simulink model "PSKs_Lab"  (R2021a)
settings: Solver=VariableStepAuto  StartTime=0.0  StopTime=50/Rb  FixedStep=1e-8  RelTol=1e-3
values from neighbouring files (symbols this model uses):
  Amplitud = 1    [Sinc_PSKm.m]
  Ancho_banda_minimo = Rb / 2    (= 500)    [Sinc_PSKm.m]
  Att_pot_Canal = 10^(Att_dB / 10)    [Sinc_PSKm.m]
  Att_Volt_Canal = 10^(Att_dB / 20)    [Sinc_PSKm.m]
  b = 0.6    [Sinc_PSKm.m]
  C = 1e-6    (= 1e-06)    [Sinc_PSKm.m]
  Frec_port = 100 * Rb    (= 100000)    [Sinc_PSKm.m]
  Kv = 1E5    (= 100000)    [Sinc_PSKm.m]
  Pot_Ruido = 2*eta * Ancho_banda_minimo    [Sinc_PSKm.m]
  R1 = Kp * Kv / (wn^2 * C)    (= 98.7654320988)    [Sinc_PSKm.m]
  R2 = 2 * zita / (wn * C)    (= 53.3333333333)    [Sinc_PSKm.m]
  Rb = 1000    [Sinc_PSKm.m]
  Retraso_Canal = Long_Canal / C_canal+0.5/Frec_port    (= 3.83333333333e-05)    [Sinc_PSKm.m]
  Tb = 1 / Rb    (= 0.001)    [Sinc_PSKm.m]
  Umbral = 0    [Sinc_PSKm.m]
libraries: dspsigops x4, dsparch4 x3, simulink_extras x3, simulink x2, commsynccomp2 x2, powerlib_extras x2, commrandsrc3 x1
settings Model: Creator=PedroPablo  LastModifiedBy=ppbot
settings SolverCC: AlgebraicLoopSolver=TrustRegion
settings DebuggingCC: SFMachineParentedDataDiag=warning

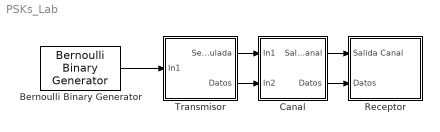
== system PSKs_Lab ==
  Bernoulli Binary Generator : commrandsrc3/Bernoulli Binary Generator  ProbabilityOfZero=0.5  SeedSource=Parameter  Seed=61  SampleTime=1/Rb  SamplesPerFrame=1  OutputDataType=double  SimulateUsing=Interpreted execution
  Canal : Subsystem
  Receptor : Subsystem
  Transmisor : Subsystem
  wires:
  Bernoulli Binary Generator/1 -> Transmisor/1(In1)
  Transmisor/1(Señal modulada) -> Canal/1(In1)
  Transmisor/2(Datos) -> Canal/2(In2)
  Canal/1(Salida Canal) -> Receptor/1(Salida Canal)
  Canal/2(Datos) -> Receptor/2(Datos)

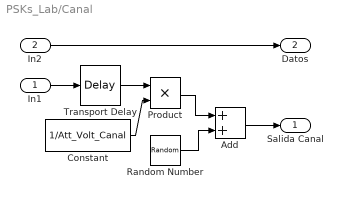
== system PSKs_Lab/Canal ==
  In1 : Inport
  In2 : Inport  Port=2
  Add : Sum
  Constant : Constant  Value=1/Att_Volt_Canal
  Product : Product
  Random Number : RandomNumber  Variance=Pot_Ruido  SampleTime=1/(10000*Rb)
  Transport Delay : TransportDelay  DelayTime=Retraso_Canal
  Salida Canal : Outport
  Datos : Outport  Port=2
  wires:
  In2/1 -> Datos/1
  Product/1 -> Add/1
  Add/1 -> Salida Canal/1
  Constant/1 -> Product/2
  In1/1 -> Transport Delay/1
  Random Number/1 -> Add/2
  Transport Delay/1 -> Product/1

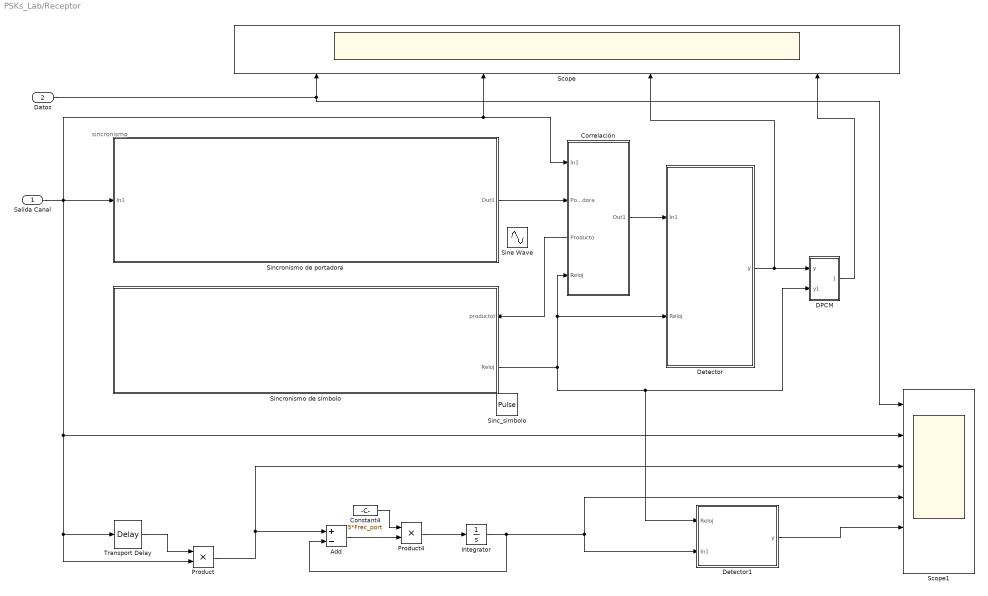
== system PSKs_Lab/Receptor ==
  note: sincronismo
  Salida Canal : Inport
  Datos : Inport  Port=2
  Add : Sum  Inputs=+-
  Constant4 : Constant  Value=5*Frec_port
  Correlación : Subsystem
      settings: PortSchema="{\"entries\":[{\"content\":{\"sides\":[{\"content\":{\"connectorIds\":[\"In1\",\"In2\",\"Out2\",\"In3\"]},\"type\":\"ConnectorPlacement.EquallySpacedRectSide\",\"uuid\":\"9c9ed9ca-e8ca-44c2-a659-85a067b2e2ab\"},{\"content\":{\"connectorIds\":[\"Out1\"],\"side\":\"RIGHT\"},\"type\":\"ConnectorPlacement.EquallySpacedRectSide\",\"uuid\":\"749548a8-d339-4a18-8c47-3529cad88115\"},{\"content\":{\"connectorIds\":[],\"side\":\"TOP\"},\"type\":\"ConnectorPlacement.EquallySpacedRectSide\",\"uuid\":\"502cb8ca-7e6c-4f6d-9acf-9edc021ca5d9\"},{\"content\":{\"connectorIds\":[],\"side\":\"BOTTOM\"},\"type\":\"ConnectorPlacement.EquallySpacedRectSide\",\"uuid\":\"343f95ab-8b43-4ca2-96bf-a55a52c277fe\"}]},\"type\":\"ConnectorPlacement.EquallySpacedConnector\",\"uuid\":\"c50381c4-8798-4039-a023-6424d6fa731c\"}],\"packageUris\":[\"http://schema.mathworks.com/mf0/Connector/R2020b\"],\"version\":\"1.0\"}"
  DPCM : Subsystem
  Detector : Subsystem
  Detector1 : Subsystem
  Integrator : Integrator
  Product : Product
  Product4 : Product
  Scope : Scope  NumInputPorts=4
  Scope1 : Scope  NumInputPorts=6
  Sinc_simbolo : DiscretePulseGenerator  PulseType=Time based  Amplitude=Amplitud  Period=1/Rb  PulseWidth=50
  Sincronismo de portadora : Subsystem
  Sincronismo de símbolo : Subsystem
      settings: PortSchema="{\"entries\":[{\"content\":{\"sides\":[{\"content\":{\"connectorIds\":[]},\"type\":\"ConnectorPlacement.EquallySpacedRectSide\",\"uuid\":\"93994b0c-b2cb-4331-9695-4cda4bbb6019\"},{\"content\":{\"connectorIds\":[\"In1\",\"Out1\"],\"side\":\"RIGHT\"},\"type\":\"ConnectorPlacement.EquallySpacedRectSide\",\"uuid\":\"b8064540-0ede-4985-840d-1e59709fa35b\"},{\"content\":{\"connectorIds\":[],\"side\":\"TOP\"},\"type\":\"ConnectorPlacement.EquallySpacedRectSide\",\"uuid\":\"0f7e7988-f1a5-40c2-b0ce-e0a51a477c0a\"}]},\"type\":\"ConnectorPlacement.EquallySpacedConnector\",\"uuid\":\"3553a0bb-71d1-453e-9ff3-b6164d2735c0\"}],\"packageUris\":[\"http://schema.mathworks.com/mf0/Connector/R2020b\"],\"version\":\"1.0\"}"
  Sine Wave : Sin  Amplitude=Amplitud/Att_Volt_Canal  Frequency=2*pi*Frec_port  SampleTime=0
  Transport Delay : TransportDelay  DelayTime=Tb
  wires:
  Datos/1 -> Scope/1, Scope1/1
  Correlación/1(Out1) -> Detector/1(In1)
  Detector/1(y) -> Scope/3, DPCM/1(y)
  Sincronismo de portadora/1(Out1) -> Correlación/2(Portadora)
  Sincronismo de símbolo/1(Reloj) -> Correlación/3(Reloj), Detector/2(Reloj), Detector1/1(Reloj), DPCM/2(y1)
  Salida Canal/1 -> Transport Delay/1, Product/2, Scope1/2, Correlación/1(In1), Scope/2, Sincronismo de portadora/1(In1)
  Correlación/2(Producto) -> Sincronismo de símbolo/1(productol)
  DPCM/1(Out1) -> Scope/4
  Transport Delay/1 -> Product/1
  Product/1 -> Scope1/3, Add/1
  Constant4/1 -> Product4/1
  Product4/1 -> Integrator/1
  Integrator/1 -> Add/2, Detector1/2(In1), Scope1/4
  Add/1 -> Product4/2
  Detector1/1(y) -> Scope1/5

== system PSKs_Lab/Transmisor ==
  In1 : Inport
  Analog Filter Design : dsparch4/Analog Filter Design  method=Butterworth  filttype=Bandpass  N=2  Wlo=2*pi*(Frec_port - 2*Ancho_banda_minimo)  Whi=2*pi*(Frec_port + 2*Ancho_banda_minimo)  Rp=2  Rs=40
  Modulador : Subsystem
  Señal modulada : Outport
  Datos : Outport  Port=2
  wires:
  In1/1 -> Modulador/1(In1), Datos/1
  Analog Filter Design/1 -> Señal modulada/1
  Modulador/1(Out1) -> Analog Filter Design/1

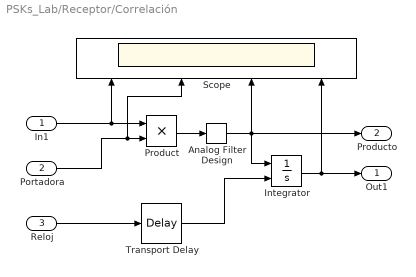
== system PSKs_Lab/Receptor/Correlación ==
  In1 : Inport
  Portadora : Inport  Port=2
  Reloj : Inport  Port=3
  Analog Filter Design : dsparch4/Analog Filter Design  method=Butterworth  filttype=Lowpass  N=8  Wlo=2*pi*Rb  Whi=80  Rp=2  Rs=40
  Integrator : Integrator  ExternalReset=rising
  Product : Product
  Scope : Scope  NumInputPorts=4
  Transport Delay : TransportDelay  DelayTime=1e-9
  Out1 : Outport
  Producto : Outport  Port=2
  wires:
  Transport Delay/1 -> Integrator/2
  In1/1 -> Product/1, Scope/1
  Integrator/1 -> Out1/1, Scope/4
  Reloj/1 -> Transport Delay/1
  Product/1 -> Analog Filter Design/1
  Portadora/1 -> Scope/2, Product/2
  Analog Filter Design/1 -> Integrator/1, Scope/3, Producto/1

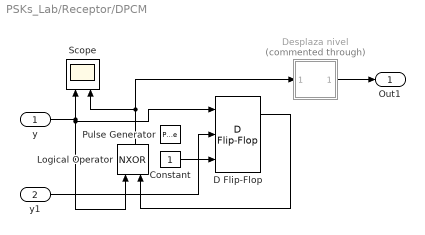
== system PSKs_Lab/Receptor/DPCM ==
  y : Inport
  y1 : Inport  Port=2
  Constant : Constant
  D Flip-Flop : simulink_extras/Flip Flops/D Flip-Flop
  Desplaza nivel : Subsystem  Commented=through
  Logical Operator : Logic  Operator=NXOR  AllPortsSameDT=off  OutDataTypeStr=boolean
  Pulse Generator : DiscretePulseGenerator  PulseType=Time based  Period=Tb
  Scope : Scope  NumInputPorts=2
  Out1 : Outport
  wires:
  Logical Operator/1 -> Desplaza nivel/1(In1), Scope/2
  D Flip-Flop/1 -> Logical Operator/2
  Constant/1 -> D Flip-Flop/3
  y/1 -> Scope/1, D Flip-Flop/1, Logical Operator/1
  Desplaza nivel/1(Out1) -> Out1/1
  y1/1 -> D Flip-Flop/2

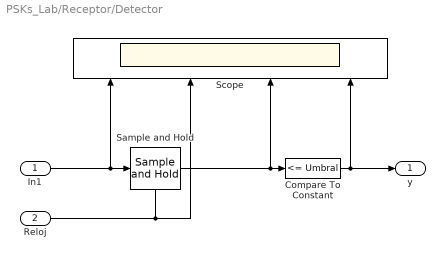
== system PSKs_Lab/Receptor/Detector ==
  In1 : Inport
  Reloj : Inport  Port=2
  Compare To Constant : simulink/Logic and Bit Operations/Compare To Constant  relop=<=  const=Umbral  OutDataTypeStr=boolean
  Sample and Hold : dspsigops/Sample and Hold  trig=Rising edge  initCond=0  latchinput=off
  Scope : Scope  NumInputPorts=4
  y : Outport
  wires:
  In1/1 -> Sample and Hold/1, Scope/1
  Compare To Constant/1 -> Scope/4, y/1
  Reloj/1 -> Scope/2, Sample and Hold/Trigger
  Sample and Hold/1 -> Scope/3, Compare To Constant/1

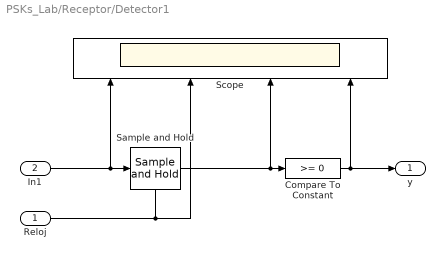
== system PSKs_Lab/Receptor/Detector1 ==
  Reloj : Inport
  In1 : Inport  Port=2
  Compare To Constant : simulink/Logic and Bit Operations/Compare To Constant  relop=>=  const=0  OutDataTypeStr=boolean
  Sample and Hold : dspsigops/Sample and Hold  trig=Rising edge  initCond=0  latchinput=off
  Scope : Scope  NumInputPorts=4
  y : Outport
  wires:
  In1/1 -> Sample and Hold/1, Scope/1
  Compare To Constant/1 -> Scope/4, y/1
  Reloj/1 -> Scope/2, Sample and Hold/Trigger
  Sample and Hold/1 -> Scope/3, Compare To Constant/1

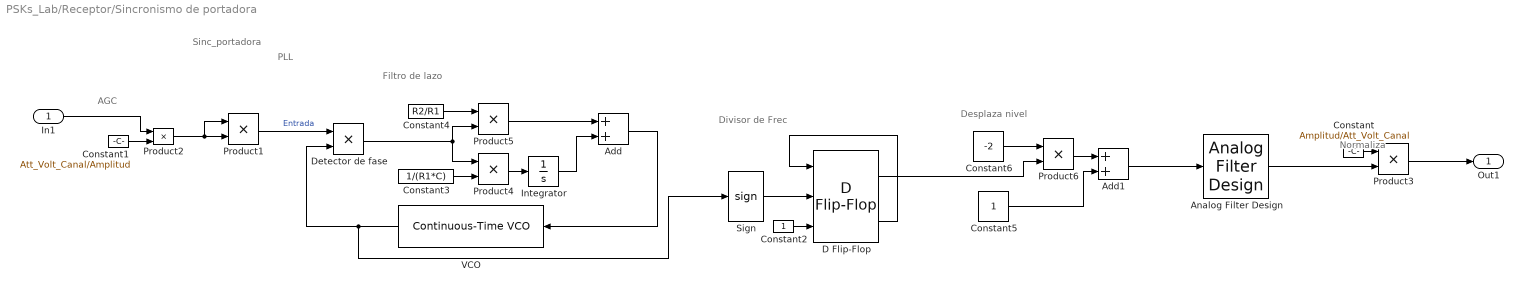
== system PSKs_Lab/Receptor/Sincronismo de portadora ==
  note: Desplaza nivel
  note: Filtro de lazo
  note: Divisor de Frec
  note: PLL
  note: Normaliza
  note: Sinc_portadora
  note: AGC
  In1 : Inport
  " VCO" : commsynccomp2/Continuous-Time VCO  Ac=1  Fc=2*Frec_port  Kc=Kv/(2*pi)  Ph=0
      settings: SourceProductBaseCode=CM
  Add : Sum
  Add1 : Sum
  Analog Filter Design : dsparch4/Analog Filter Design  method=Butterworth  filttype=Bandpass  N=2  Wlo=1.8*pi*Frec_port  Whi=2.2*pi*Frec_port  Rp=2  Rs=40
  Constant : Constant  Value=Amplitud/Att_Volt_Canal
  Constant1 : Constant  Value=Att_Volt_Canal/Amplitud
  Constant2 : Constant
  Constant3 : Constant  Value=1/(R1*C)
  Constant4 : Constant  Value=R2/R1
  Constant5 : Constant
  Constant6 : Constant  Value=-2
  D Flip-Flop : simulink_extras/Flip Flops/D Flip-Flop
  Detector de fase : Product
  Integrator : Integrator
  Product{1..6} (6 alike) : Product
  Sign : Signum
  Out1 : Outport
  wires:
  Product3/1 -> Out1/1
  In1/1 -> Product2/1
  Constant1/1 -> Product2/2
  Product2/1 -> Product1/1, Product1/2
  Constant/1 -> Product3/1
  Add1/1 -> Analog Filter Design/1
  Add/1 -> " VCO"/1
  Product1/1 -> Detector de fase/1  "Entrada"
  Sign/1 -> D Flip-Flop/2
  " VCO"/1 -> Detector de fase/2, Sign/1
  D Flip-Flop/2 -> D Flip-Flop/1
  Constant2/1 -> D Flip-Flop/3
  Constant4/1 -> Product5/1
  Product5/1 -> Add/1
  Detector de fase/1 -> Product5/2, Product4/1
  Product4/1 -> Integrator/1
  Integrator/1 -> Add/2
  Constant3/1 -> Product4/2
  Constant5/1 -> Add1/2
  Product6/1 -> Add1/1
  Constant6/1 -> Product6/1
  D Flip-Flop/1 -> Product6/2
  Analog Filter Design/1 -> Product3/2

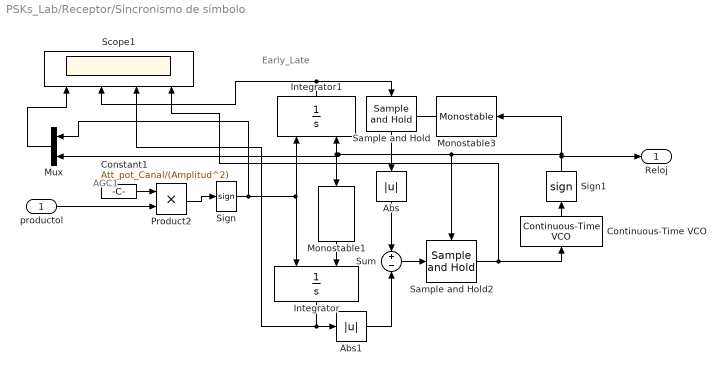
== system PSKs_Lab/Receptor/Sincronismo de símbolo ==
  note: Early_Late
  note: AGC1
  productol : Inport
  Abs : Abs
  Abs1 : Abs
  Constant1 : Constant  Value=Att_pot_Canal/(Amplitud^2)
  Continuous-Time VCO : commsynccomp2/Continuous-Time VCO  Ac=1  Fc=Rb  Kc=kv2  Ph=1.75*pi
      settings: SourceProductBaseCode=CM
  Integrator : Integrator  ExternalReset=falling  UpperSaturationLimit=0.7e-4  LowerSaturationLimit=-0.7e-4
  Integrator1 : Integrator  ExternalReset=rising  UpperSaturationLimit=0.7e-4  LowerSaturationLimit=-0.7e-4
  Monostable1 : powerlib_extras/Control  Blocks/Monostable  EdgeDetect=Rising  t_mono=(1-b)/Rb  ic=0
      settings: SourceProductBaseCode=PS
  Monostable3 : powerlib_extras/Control  Blocks/Monostable  EdgeDetect=Rising  t_mono=b/Rb  ic=0
      settings: SourceProductBaseCode=PS
  Mux : Mux  Inputs=2
  Product2 : Product
  Sample and Hold : dspsigops/Sample and Hold  trig=Falling edge  initCond=0  latchinput=off
  Sample and Hold2 : dspsigops/Sample and Hold  trig=Rising edge  initCond=0  latchinput=off
  Scope1 : Scope  NumInputPorts=4
  Sign : Signum
  Sign1 : Signum
  Sum : Sum  Inputs=+-
  Reloj : Outport
  wires:
  Sign1/1 -> Monostable3/1, Mux/2, Monostable1/1, Integrator1/2, Sample and Hold2/Trigger, Reloj/1
  Product2/1 -> Sign/1
  Constant1/1 -> Product2/1
  productol/1 -> Product2/2
  Sign/1 -> Integrator/1, Integrator1/1, Mux/1
  Continuous-Time VCO/1 -> Sign1/1
  Abs/1 -> Sum/1
  Sum/1 -> Sample and Hold2/1
  Integrator1/1 -> Sample and Hold/1, Scope1/2
  Abs1/1 -> Sum/2
  Sample and Hold/1 -> Abs/1
  Integrator/1 -> Scope1/3, Abs1/1
  Monostable3/1 -> Sample and Hold/Trigger
  Monostable1/1 -> Integrator/2
  Sample and Hold2/1 -> Continuous-Time VCO/1, Scope1/4
  Mux/1 -> Scope1/1

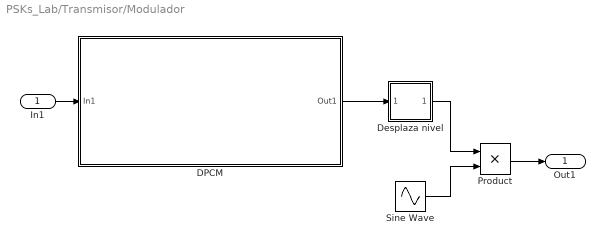
== system PSKs_Lab/Transmisor/Modulador ==
  In1 : Inport
  DPCM : Subsystem
  Desplaza nivel : Subsystem
  Product : Product
  Sine Wave : Sin  Amplitude=Amplitud  Frequency=2*pi*(Frec_port)  SampleTime=0
  Out1 : Outport
  wires:
  Sine Wave/1 -> Product/2
  Product/1 -> Out1/1
  Desplaza nivel/1(Out1) -> Product/1
  In1/1 -> DPCM/1(In1)
  DPCM/1(Out1) -> Desplaza nivel/1(In1)

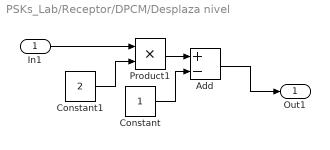
== system PSKs_Lab/Receptor/DPCM/Desplaza nivel ==
  In1 : Inport
  Add : Sum  Inputs=+-
  Constant : Constant
  Constant1 : Constant  Value=2
  Product1 : Product
  Out1 : Outport
  wires:
  In1/1 -> Product1/1
  Product1/1 -> Add/1
  Constant1/1 -> Product1/2
  Constant/1 -> Add/2
  Add/1 -> Out1/1

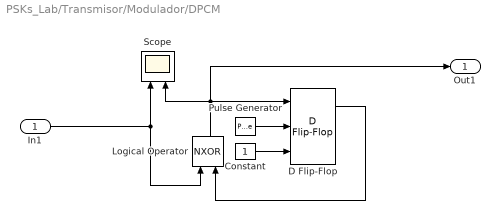
== system PSKs_Lab/Transmisor/Modulador/DPCM ==
  In1 : Inport
  Constant : Constant
  D Flip-Flop : simulink_extras/Flip Flops/D Flip-Flop
  Logical Operator : Logic  Operator=NXOR  AllPortsSameDT=off  OutDataTypeStr=boolean
  Pulse Generator : DiscretePulseGenerator  PulseType=Time based  Period=Tb  PulseWidth=50
  Scope : Scope  NumInputPorts=2
  Out1 : Outport
  wires:
  In1/1 -> Logical Operator/1, Scope/1
  Logical Operator/1 -> Out1/1, D Flip-Flop/1, Scope/2
  D Flip-Flop/1 -> Logical Operator/2
  Pulse Generator/1 -> D Flip-Flop/2
  Constant/1 -> D Flip-Flop/3

== system PSKs_Lab/Transmisor/Modulador/Desplaza nivel ==
  In1 : Inport
  Add : Sum  Inputs=+-
  Constant : Constant
  Constant1 : Constant  Value=2
  Product1 : Product
  Out1 : Outport
  wires:
  In1/1 -> Product1/1
  Product1/1 -> Add/1
  Constant1/1 -> Product1/2
  Constant/1 -> Add/2
  Add/1 -> Out1/1
